simulink model "StPassCmprtMdHMIDisCmd"  (R2018b)
settings: Solver=FixedStepDiscrete  StartTime=0.0  StopTime=10.0  FixedStep=0.01  RelTol=1e-3
undefined symbols (not defined in the file or in its folder): PowerMode1
libraries: RspLib x1
settings Model: Creator=sn2xws  LastModifiedBy=sn2xws
settings DataIOCC: SaveFormat=StructureWithTime
settings OptimizationCC: DefaultParameterBehavior=Inlined  EnhancedBackFolding=on  PassReuseOutputArgsAs=Individual arguments  ZeroExternalMemoryAtStartup=off  ZeroInternalMemoryAtStartup=off  OptimizeBlockOrder=speed  DifferentSizesBufferReuse=on  OptimizationCustomize=off
settings DebuggingCC: ParameterTunabilityLossMsg=error
settings ModelReferenceCC: ModelReferenceNumInstancesAllowed=Single
settings SFSimCC: MATLABDynamicMemAlloc=off
settings RTWCC: SystemTargetFile=autosar.tlc  GenCodeOnly=on  TemplateMakefile=ert_default_tmf  Description=AUTOSAR  GenerateReport=on  IncludeHyperlinkInReport=on  LaunchReport=on  GenerateTraceInfo=on  GenerateTraceReport=on  GenerateTraceReportSl=on  GenerateTraceReportSf=on  GenerateTraceReportEml=on  GenerateCodeMetricsReport=on
settings CodeAppCC: ForceParamTrailComments=on  IgnoreCustomStorageClasses=off  OperatorAnnotations=on  SimulinkDataObjDesc=on  SFDataObjDesc=on  InsertBlockDesc=on
settings STFCustomTargetCC: TargetLangStandard=C99 (ISO)  MultiwordLength=256  ParMdlRefBuildCompliant=on  CompOptLevelCompliant=on  IncludeMdlTerminateFcn=off  CombineOutputUpdateFcns=on  SuppressErrorStatus=on  ERTCustomFileBanners=on  SupportNonFinite=off  SupportComplex=off  SupportContinuousTime=off  SupportNonInlinedSFcns=off  RemoveResetFunc=on  MATLABClassNameForMDSCustomization=Simulink.SoftwareTarget.ERTCustomization  AutosarCompliant=on  UseToolchainInfoCompliant=on  LookupTableObjectStructAxisOrder=2,1,3,4,...  LUTObjectStructOrderEvenSpacing=Size,Table,Breakpoints  SystemTargetFile=autosar.tlc
settings ERTTargetCC: TargetLangStandard=C99 (ISO)  ConcurrentExecutionCompliant=off  IncludeMdlTerminateFcn=off  SuppressErrorStatus=on  SupportNonFinite=off  SupportComplex=off  ModelStepFunctionPrototypeControlCompliant=off  CPPClassGenCompliant=off  AutosarCompliant=on  LookupTableObjectStructAxisOrder=2,1,3,4,...  LUTObjectStructOrderEvenSpacing=Size,Table,Breakpoints  InlinedParameterPlacement=NonHierarchical  ERTCustomFileTemplate=example_file_process.tlc  ERTFilePackagingFormat=Compact

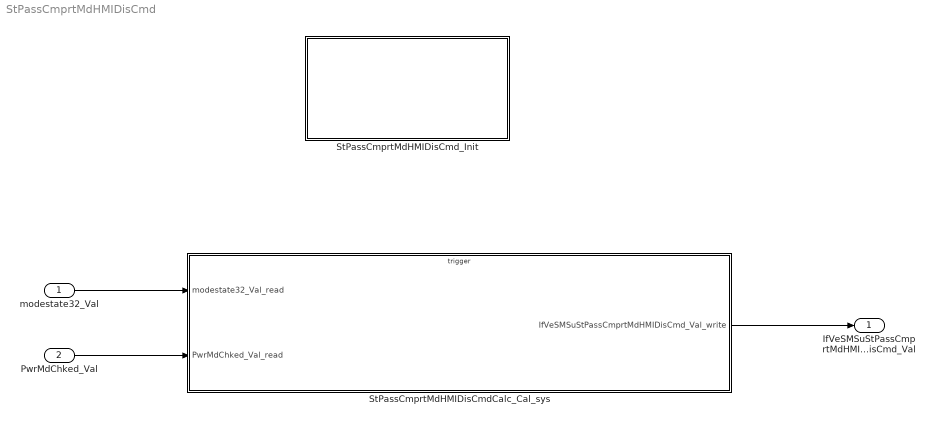
== system StPassCmprtMdHMIDisCmd ==
  modestate32_Val : Inport  OutDataTypeStr=uint32  PortDimensions=1
  PwrMdChked_Val : Inport  Port=2  OutDataTypeStr=Enum: PowerMode1  PortDimensions=1
  StPassCmprtMdHMIDisCmdCalc_Cal_sys : Subsystem
  StPassCmprtMdHMIDisCmd_Init : Subsystem
  IfVeSMSuStPassCmprtMdHMIDisCmd_Val : Outport  OutDataTypeStr=uint8  PortDimensions=1
  wires:
  modestate32_Val/1 -> StPassCmprtMdHMIDisCmdCalc_Cal_sys/1(modestate32_Val_read)
  PwrMdChked_Val/1 -> StPassCmprtMdHMIDisCmdCalc_Cal_sys/2(PwrMdChked_Val_read)
  StPassCmprtMdHMIDisCmdCalc_Cal_sys/1(IfVeSMSuStPassCmprtMdHMIDisCmd_Val_write) -> IfVeSMSuStPassCmprtMdHMIDisCmd_Val/1

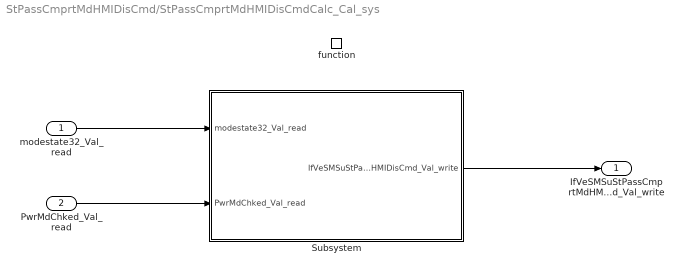
== system StPassCmprtMdHMIDisCmd/StPassCmprtMdHMIDisCmdCalc_Cal_sys ==
  modestate32_Val_read : Inport
  PwrMdChked_Val_read : Inport  Port=2
  function : TriggerPort  TriggerType=function-call  IsSimulinkFunction=on  FunctionName=StPassCmprtMdHMIDisCmdCalc_Cal  VariantControl=(inherit)
  Subsystem : Subsystem
  IfVeSMSuStPassCmprtMdHMIDisCmd_Val_write : Outport
      settings: EnsureOutportIsVirtual=on
  wires:
  modestate32_Val_read/1 -> Subsystem/1(modestate32_Val_read)
  PwrMdChked_Val_read/1 -> Subsystem/2(PwrMdChked_Val_read)
  Subsystem/1(IfVeSMSuStPassCmprtMdHMIDisCmd_Val_write) -> IfVeSMSuStPassCmprtMdHMIDisCmd_Val_write/1

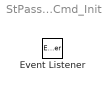
== system StPassCmprtMdHMIDisCmd/StPassCmprtMdHMIDisCmd_Init ==
  Event Listener : EventListener  EventName=reset

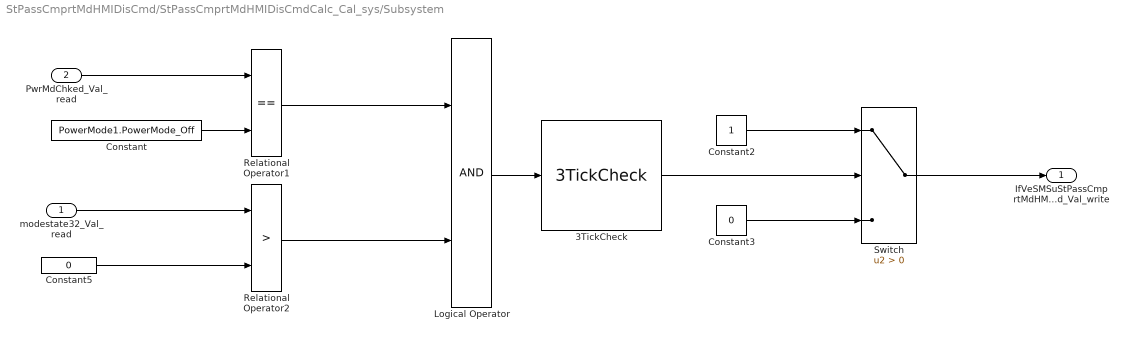
== system StPassCmprtMdHMIDisCmd/StPassCmprtMdHMIDisCmdCalc_Cal_sys/Subsystem ==
  modestate32_Val_read : Inport
  PwrMdChked_Val_read : Inport  Port=2
  3TickCheck : RspLib/3TickCheck  SystemSampleTime=-1
  Constant : Constant  Value=PowerMode1.PowerMode_Off  OutDataTypeStr=Enum:PowerMode1
  Constant2 : Constant  OutDataTypeStr=uint8
  Constant3 : Constant  Value=0  OutDataTypeStr=uint8
  Constant5 : Constant  Value=0  OutDataTypeStr=uint32
  Logical Operator : Logic  AllPortsSameDT=off  OutDataTypeStr=boolean
  Relational Operator1 : RelationalOperator  Operator===  OutDataTypeStr=boolean  RndMeth=Simplest
  Relational Operator2 : RelationalOperator  Operator=>  OutDataTypeStr=boolean  RndMeth=Simplest
  Switch : Switch  Criteria=u2 > Threshold
  IfVeSMSuStPassCmprtMdHMIDisCmd_Val_write : Outport
      settings: EnsureOutportIsVirtual=on
  wires:
  Switch/1 -> IfVeSMSuStPassCmprtMdHMIDisCmd_Val_write/1
  modestate32_Val_read/1 -> Relational Operator2/1
  Constant5/1 -> Relational Operator2/2
  Constant2/1 -> Switch/1
  Constant/1 -> Relational Operator1/2
  3TickCheck/1 -> Switch/2
  Constant3/1 -> Switch/3
  Logical Operator/1 -> 3TickCheck/1
  Relational Operator1/1 -> Logical Operator/1
  Relational Operator2/1 -> Logical Operator/2
  PwrMdChked_Val_read/1 -> Relational Operator1/1
